simulink model "Openended1"  (R2025b)
settings: Solver=VariableStepAuto  StartTime=0.0  StopTime=2.0  RelTol=1e-3

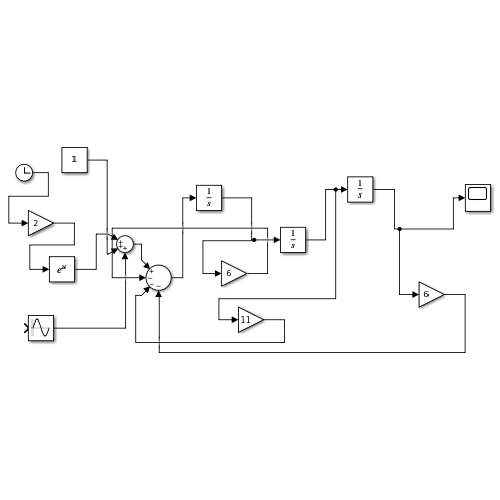
[thumbnail: Simulink's stored preview of the top-level diagram]
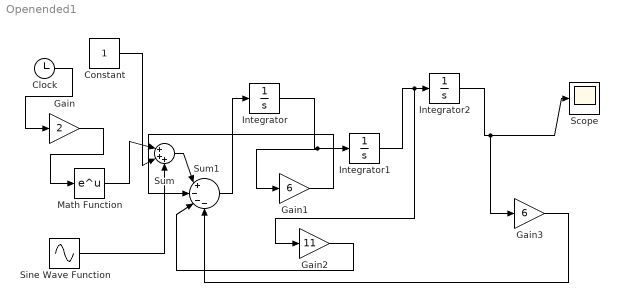
== system Openended1 ==
  Clock : Clock
  Constant : Constant
  Gain : Gain  Gain=2
  Gain1 : Gain  Gain=6
  Gain2 : Gain  Gain=11
  Gain3 : Gain  Gain=6
  Integrator : Integrator  InitialCondition=2
  Integrator1 : Integrator  InitialCondition=1
  Integrator2 : Integrator  InitialCondition=1
  Math Function : Math
  Scope : Scope
      settings: ActiveDisplayYMinimum=0.90962471649315235  ActiveDisplayYMaximum=1.8133775515616297
  Sine Wave Function : Sin  TimeSource=Use external signal  SampleTime=0
  Sum : Sum  Inputs=|+++
  Sum1 : Sum  Inputs=|+---
  wires:
  Clock/1 -> Gain/1
  Gain/1 -> Math Function/1
  Constant/1 -> Sum/2
  Math Function/1 -> Sum/1
  Sine Wave Function/1 -> Sum/3
  Sum/1 -> Sum1/1
  Sum1/1 -> Integrator/1
  Integrator/1 -> Gain1/1, Integrator1/1
  Integrator1/1 -> Gain2/1, Integrator2/1
  Integrator2/1 -> Scope/1, Gain3/1
  Gain3/1 -> Sum1/4
  Gain2/1 -> Sum1/3
  Gain1/1 -> Sum1/2
